simulink model "sim_par_calculado"  (R2019b)
settings: Solver=ode4  StartTime=0.0  StopTime=40.0  FixedStep=0.005  RelTol=1e-3
values from neighbouring files (symbols this model uses):
  Kp = [kp 0;         0 kp]    [par_calculado.m]
  Kv = [kv 0;         0 kv]    [par_calculado.m]
  q0 = [90*pi/180;0*pi/180;0;0]    [par_calculado.m]    (also in slotine_li.m = [90*pi/180;0;0;0])
  theta = load('../theta.mat').theta    [par_calculado.m]    (also in slotine_li.m)
settings Model: Creator=AlejnadroZapett  LastModifiedBy=AlejnadroZapett

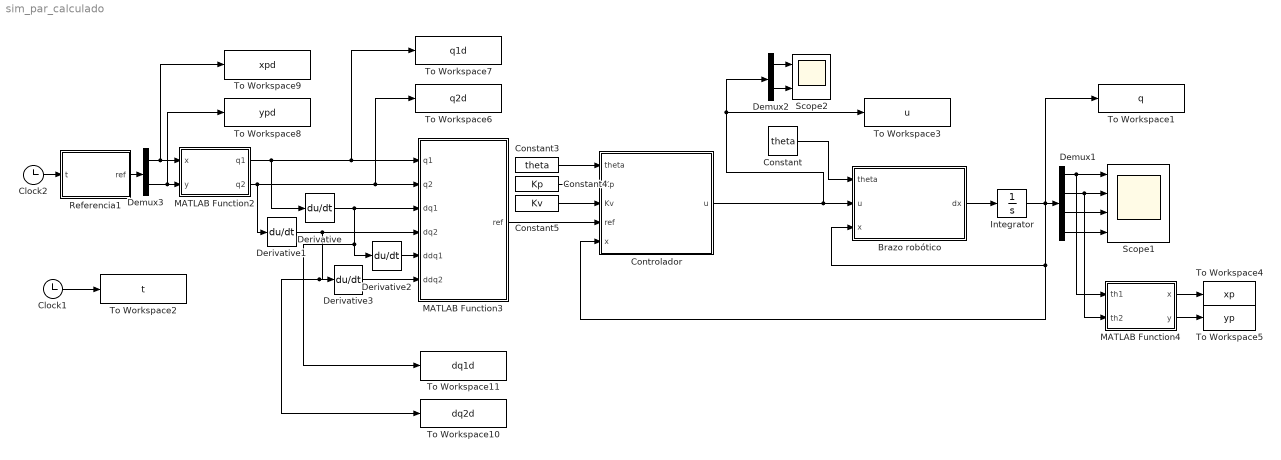
== system sim_par_calculado ==
  Brazo robótico : MATLAB Function  TreatAsAtomicUnit=on
  Clock1 : Clock
  Clock2 : Clock
  Constant : Constant  Value=theta
  Constant3 : Constant  Value=theta
  Constant4 : Constant  Value=Kp
  Constant5 : Constant  Value=Kv
  Controlador : MATLAB Function  TreatAsAtomicUnit=on
  Demux1 : Demux
  Demux2 : Demux  Outputs=2
  Demux3 : Demux  Outputs=2
  Derivative{,1..3} (4 alike) : Derivative
  Integrator : Integrator  InitialCondition=q0
  MATLAB Function2 : MATLAB Function  TreatAsAtomicUnit=on
  MATLAB Function3 : MATLAB Function  TreatAsAtomicUnit=on
  MATLAB Function4 : MATLAB Function  TreatAsAtomicUnit=on
  Referencia1 : MATLAB Function  TreatAsAtomicUnit=on
  Scope1 : Scope  NumInputPorts=4
  Scope2 : Scope  NumInputPorts=2
  To Workspace1 : ToWorkspace  VariableName=q  SampleTime=-1
  To Workspace10 : ToWorkspace  VariableName=dq2d  SampleTime=-1
  To Workspace11 : ToWorkspace  VariableName=dq1d  SampleTime=-1
  To Workspace2 : ToWorkspace  VariableName=t  SampleTime=-1
  To Workspace3 : ToWorkspace  VariableName=u  SampleTime=-1
  To Workspace4 : ToWorkspace  VariableName=xp  SampleTime=-1
  To Workspace5 : ToWorkspace  VariableName=yp  SampleTime=-1
  To Workspace6 : ToWorkspace  VariableName=q2d  SampleTime=-1
  To Workspace7 : ToWorkspace  VariableName=q1d  SampleTime=-1
  To Workspace8 : ToWorkspace  VariableName=ypd  SampleTime=-1
  To Workspace9 : ToWorkspace  VariableName=xpd  SampleTime=-1
  wires:
  Integrator/1 -> To Workspace1/1, Demux1/1, Controlador/5(x), Brazo robótico/3(x)
  Demux1/2 -> MATLAB Function4/2(th2), Scope1/2
  Demux1/1 -> MATLAB Function4/1(th1), Scope1/1
  Constant/1 -> Brazo robótico/1(theta)
  Demux2/2 -> Scope2/2
  Demux1/3 -> Scope1/3
  Demux1/4 -> Scope1/4
  Clock1/1 -> To Workspace2/1
  Brazo robótico/1(dx) -> Integrator/1
  Demux2/1 -> Scope2/1
  Constant3/1 -> Controlador/1(theta)
  Constant4/1 -> Controlador/2(Kp)
  Constant5/1 -> Controlador/3(Kv)
  Demux3/1 -> To Workspace9/1, MATLAB Function2/1(x)
  Clock2/1 -> Referencia1/1(t)
  Referencia1/1(ref) -> Demux3/1
  Demux3/2 -> To Workspace8/1, MATLAB Function2/2(y)
  MATLAB Function3/1(ref) -> Controlador/4(ref)
  MATLAB Function2/1(q1) -> To Workspace7/1, MATLAB Function3/1(q1), Derivative/1
  MATLAB Function2/2(q2) -> Derivative1/1, To Workspace6/1, MATLAB Function3/2(q2)
  Derivative/1 -> To Workspace11/1, Derivative2/1, MATLAB Function3/3(dq1)
  Derivative1/1 -> To Workspace10/1, Derivative3/1, MATLAB Function3/4(dq2)
  Derivative2/1 -> MATLAB Function3/5(ddq1)
  Derivative3/1 -> MATLAB Function3/6(ddq2)
  MATLAB Function4/1(x) -> To Workspace4/1
  MATLAB Function4/2(y) -> To Workspace5/1
  Controlador/1(u) -> To Workspace3/1, Demux2/1, Brazo robótico/2(u)

== matlab function sim_par_calculado/Brazo robótico ==
  data: theta input; u input; dx output; x input
function dx = fcn(theta,u,x)

dx = zeros(4,1);

u1 = u(1);
u2 = u(2);

q1 = x(1);
q2 = x(2);
dq1 = x(3);
dq2 = x(4);

M11 = (theta(1) + theta(2)*cos(q1));
M12 = (theta(3) + theta(4)*cos(q2));
M21 = (theta(11) + theta(12)*cos(q2));
M22 = theta(13);

C11 = theta(5)*sin(q2)*dq2;
C12 = theta(6)*sin(q2)*dq2;
C21 = theta(14)*sin(q2)*dq1;
C22 = 0;

G1 = theta(7)*cos(q1)+theta(8)*cos(q1+q2);
G2 = theta(14)*cos(q1+q2);

% F1 = theta(9)*dq1 + theta(10)*sign(dq1);
% F2 = theta(16)*dq2 + theta(17)*sign(dq2);
F1 = theta(9)*dq1;
F2 = theta(16)*dq2;

M = [M11 M12;M21 M22];
C = [C11 C12;C21 C22];
G = [G1;G2];
F = [F1;F2];
T = [u1;u2];

D = -inv(M)*(C*[dq1;dq2]+G+F-T);

dx(1) = dq1;
dx(2) = dq2;
dx(3) = D(1);
dx(4) = D(2);

== matlab function sim_par_calculado/Controlador ==
  data: theta input; Kp input; Kv input; ref input; u output; x input
function u = fcn(theta,Kp,Kv,ref,x)

q1d = ref(1);
q2d = ref(2);

dq1d = ref(3);
dq2d = ref(4);

ddq1d = ref(5);
ddq2d = ref(6);

u = zeros(2,1);

q1 = x(1);
q2 = x(2);
dq1 = x(3);
dq2 = x(4);

ddqd = [ddq1d;      ...
        ddq2d];

dq_ = [dq1d-dq1;    ...
       dq2d-dq2];
   
q_ = [q1d-q1;       ...
      q2d-q2];

M11 = (theta(1) + theta(2)*cos(q1));
M12 = (theta(3) + theta(4)*cos(q2));
M21 = (theta(11) + theta(12)*cos(q2));
M22 = theta(13);

C11 = theta(5)*sin(q2)*dq2;
C12 = theta(6)*sin(q2)*dq2;
C21 = theta(14)*sin(q2)*dq1;
C22 = 0;

G1 = theta(7)*cos(q1)+theta(8)*cos(q1+q2);
G2 = theta(14)*cos(q1+q2);

% F1 = theta(9)*dq1 + theta(10)*sign(dq1);
% F2 = theta(16)*dq2 + theta(17)*sign(dq2);
F1 = theta(9)*dq1;
F2 = theta(16)*dq2;

M = [M11 M12;M21 M22];
C = [C11 C12;C21 C22];
G = [G1;G2];
F = [F1;F2];

u = M*(ddqd + Kv*dq_ + Kp*q_)+C*[dq1;dq2]+G+F;

== matlab function sim_par_calculado/MATLAB Function2 ==
  data: x input; q1 output; y input; q2 output
function [q1,q2] = c_inv(x,y)

l1 = 0.12;
l2 = 0.14;

r=sqrt(x^2+y^2);
alfa=atan2(y,x);
beta=acos((l1^2+l2^2-r^2)/(2*l1*l2));
gama=acos((l1^2-l2^2+r^2)/(2*l1*r));
% solución codo abajo
% th1a=alfa-gama;
% th2a=pi-beta;
% solución codo arriba
th1b=alfa+gama;
th2b=pi+beta;
%q=[th1b,th2b];
q1=th1b;
q2=th2b-2*pi;

== matlab function sim_par_calculado/Referencia1 ==
  data: t input; ref output
function ref = fcn(t)

% Tiempo de duración de cada sección
t1 = 10;
t2 = 10;
t3 = 10;
t4 = 10;

% Coordenadas x,y
p_x = [0.05,0.09,0.09,0.05];
p_y = [0.24,0.24,0.20,0.20];

x = 0;
y = 5;

if t <= t1 % 1-2
    
    Po = p_x(1);
    Pf = p_x(2);
    
    ti = t;
    
    lambda = (10/(t1^3))*ti^3 - (15/(t1^4))*ti^4 + (6/(t1^5))*ti^5;
    
    x = Po + lambda*(Pf-Po);
    y = p_y(1);
    
elseif t > t1 & t <= (t1+t2) % 2-3
    
    Po = p_y(2);
    Pf = p_y(3);
    
    ti = t - t1;
    
    lambda = (10/(t2^3))*ti^3 - (15/(t2^4))*ti^4 + (6/(t2^5))*ti^5;
    
    y = Po + lambda*(Pf-Po);
    x = p_x(2);
    
elseif t > (t1+t2) & t <= (t1+t2+t3) % 3-4
    
    Po = p_x(3);
    Pf = p_x(4);
    
    ti = t -(t1+t2);
    
    lambda = (10/(t3^3))*ti^3 - (15/(t3^4))*ti^4 + (6/(t3^5))*ti^5;
    
    x = Po + lambda*(Pf-Po);
    y = p_y(4);
    
elseif t > (t1+t2+t3) & t <= (t1+t2+t3+t4) % 4-1
    
    Po = p_y(4);
    Pf = p_y(1);
    
    ti = t -(t1+t2+t3);
    
    lambda = (10/(t4^3))*ti^3 - (15/(t4^4))*ti^4 + (6/(t4^5))*ti^5;
    
    y = Po + lambda*(Pf-Po);
    x = p_x(4);
end

ref = [x;y];

== matlab function sim_par_calculado/MATLAB Function3 ==
  data: q1 input; ref output; q2 input; dq1 input; dq2 input; ddq1 input; ddq2 input
function ref = c_inv(q1,q2,dq1,dq2,ddq1,ddq2)

ref = [q1;q2;dq1;dq2;ddq1;ddq2];

== matlab function sim_par_calculado/MATLAB Function4 ==
  data: th1 input; x output; th2 input; y output
function [x,y] = c_dir(th1,th2)

l1 = 0.12;
l2 = 0.14;

px=l1*cos(th1)+l2*cos(th1+th2);
py=l1*sin(th1)+l2*sin(th1+th2);
%p=[px,py];

x=px;
y=py;
